simulink model "atrias_system_testing_delay"  (R2014a)
settings: Solver=FixedStepDiscrete  StartTime=0.0  StopTime=inf  FixedStep=sample_time  RelTol=1e-3
PreLoadFcn:
  | set_sampletime
PostLoadFcn:
  | set_sampletime
InitFcn:
  | sys_params
StartFcn:
  | set_sampletime
values from neighbouring files (symbols this model uses):
  A_lpf_velocity = 1 + B1_lpf_velocity + B2_lpf_velocity    [daq_params_osu.m]
  B1_lpf_velocity = -2*exp(-lpf_damping*fcut_velocity*sample_time)*cos(fcut_velocity*sample_time*sqrt(1-lpf_damping^2))    [daq_params_osu.m]
  B2_lpf_velocity = exp(-2*lpf_damping*fcut_velocity*sample_time)    [daq_params_osu.m]
  BOOM_MAX_ENCODER_TICKS = 2^17 - 1    (= 131071)    [daq_params_osu.m]
  BOOM_PITCH_CAL_VALUE_RAD = 0    [daq_params_osu.m]
  BOOM_PITCH_CAL_VALUE_TICKS = 43809    [daq_params_osu.m]
  BOOM_PITCH_ENCODER_RAD_PER_TICK = -2*pi / (2^17 * 2)    (= -2.39684498107e-05)    [daq_params_osu.m]
  BOOM_ROLL_CAL_VALUE_RAD = 0.1271    [daq_params_osu.m]
  BOOM_ROLL_CAL_VALUE_TICKS = 9318    [daq_params_osu.m]
  BOOM_ROLL_ENCODER_RAD_PER_TICK = 2*pi / (2^17 * 7)    (= 6.84812851735e-06)    [daq_params_osu.m]
  BOOM_YAW_ENCODER_RAD_PER_TICK = 2*pi / (2^17 * 9.6)    (= 4.9934270439e-06)    [daq_params_osu.m]
  CURRENT_LIMIT = 100    [daq_params_osu.m]
  fcut_smooth = 16*(2*pi)    (= 100.530964915)    [daq_params_osu.m]
  fcut_unwrap = 8*(2*pi)    (= 50.2654824574)    [daq_params_osu.m]
  gui_disable_cmd = 0    [daq_params_osu.m]
  gui_enable_cmd = 0    [daq_params_osu.m]
  gui_estop_cmd = 0    [daq_params_osu.m]
  gui_reset_cmd = 0    [daq_params_osu.m]
  HIP_ABS_ENCODER_RAD_PER_TICK = 2*pi / 2^13    (= 0.000766990393943)    [daq_params_osu.m]
  HIP_ABS_MAX_ENCODER_TICKS = 2^13 - 1    (= 8191)    [daq_params_osu.m]
  HIP_INC_ENCODER_RAD_PER_TICK = 2*pi / (2500 * 4 * 57)    (= 1.10231321179e-05)    [daq_params_osu.m]
  HIP_INC_MAX_ENCODER_TICKS = 2^16 - 1    (= 65535)    [daq_params_osu.m]
  HIP_MOTOR_CONSTANT = 0.184    [daq_params_osu.m]
  HIP_MTR_GEAR_RATIO = 57    [daq_params_osu.m]
  HIP_MTR_MAX_TORQUE = MTR_HIP_MAX_CURRENT*HIP_MOTOR_CONSTANT*HIP_MTR_GEAR_RATIO    (= 629.28)    [daq_params_osu.m]
  INC_ENC_DIRS = -[ LEG1_MOTOR_A_DIRECTION ... (first row only)    [daq_params_osu.m]
  INC_ENC_RAD_PER_TICK = 2*pi/14000/LEG_MTR_GEAR_RATIO    (= 8.97597901026e-06)    [daq_params_osu.m]
  k_sea = 4118    [sys_params.m]
  LEFT_HIP_CALIB_POS = 0    [daq_params_osu.m]
  LEFT_HIP_CALIB_VAL = 7192 - 2^13    (= -1000)    [daq_params_osu.m]
  LEFT_MOTOR_HIP_DIRECTION = -1.0    (= -1)    [daq_params_osu.m]
  LEG1_LEG_A_CALIB_VAL = 265417675    [daq_params_osu.m]
  LEG1_LEG_A_RAD_PER_CNT = -9.8039216e-09    [daq_params_osu.m]
  LEG1_LEG_B_CALIB_VAL = 175319150    [daq_params_osu.m]
  LEG1_LEG_B_RAD_PER_CNT = -9.8039216e-09    [daq_params_osu.m]
  LEG1_MOTOR_A_DIRECTION = -1.0    (= -1)    [daq_params_osu.m]
  LEG1_MOTOR_B_DIRECTION = -1.0    (= -1)    [daq_params_osu.m]
  LEG1_TRAN_A_CALIB_VAL = 143046540    [daq_params_osu.m]
  LEG1_TRAN_A_RAD_PER_CNT = 9.8039216e-09    [daq_params_osu.m]
  LEG1_TRAN_B_CALIB_VAL = 142356572    [daq_params_osu.m]
  LEG1_TRAN_B_RAD_PER_CNT = -9.8039216e-09    [daq_params_osu.m]
  LEG2_LEG_A_CALIB_VAL = 264357825    [daq_params_osu.m]
  LEG2_LEG_A_RAD_PER_CNT = -9.8039216e-09    [daq_params_osu.m]
  LEG2_LEG_B_CALIB_VAL = 261444054    [daq_params_osu.m]
  LEG2_LEG_B_RAD_PER_CNT = 9.8039216e-09    [daq_params_osu.m]
  LEG2_MOTOR_A_DIRECTION = 1.0    (= 1)    [daq_params_osu.m]
  LEG2_MOTOR_B_DIRECTION = 1.0    (= 1)    [daq_params_osu.m]
  LEG2_TRAN_A_CALIB_VAL = 142300933    [daq_params_osu.m]
  LEG2_TRAN_A_RAD_PER_CNT = 9.8039216e-09    [daq_params_osu.m]
  LEG2_TRAN_B_CALIB_VAL = 142287413    [daq_params_osu.m]
  LEG2_TRAN_B_RAD_PER_CNT = -9.8039216e-09    [daq_params_osu.m]
  LEG_A_CALIB_LOC = pi + 0.305432619099008    (= 3.44702527269)    [daq_params_osu.m]
  LEG_B_CALIB_LOC = pi - 0.305432619099008    (= 2.83616003449)    [daq_params_osu.m]
  LEG_MOTOR_CONSTANT = 0.119    [daq_params_osu.m]
  LEG_MTR_GEAR_RATIO = 50    [daq_params_osu.m]
  LEG_MTR_MAX_TORQUE = MTR_MAX_CURRENT*LEG_MOTOR_CONSTANT*LEG_MTR_GEAR_RATIO    (= 922.25)    [daq_params_osu.m]
  max_encoder_velocity = 200    [daq_params_osu.m]
  MEDULLA_ADC_MAX_VOLTS = 2.70    (= 2.7)    [daq_params_osu.m]
  MEDULLA_ADC_OFFSET_COUNTS = 172    [daq_params_osu.m]
  MEDULLA_STATE_ERROR = 5    [daq_params_osu.m]
  MEDULLA_STATE_HALT = 4    [daq_params_osu.m]
  MEDULLA_STATE_IDLE = 0    [daq_params_osu.m]
  MEDULLA_STATE_RESET = 6    [daq_params_osu.m]
  MEDULLA_STATE_RUN = 2    [daq_params_osu.m]
  MEDULLA_TIMER_FREQ = 32e6    (= 32000000)    [daq_params_osu.m]
  MOTOR_POSITION_LIMITS_LOWER = [2.5; 1.4; 0.4]    [daq_params_osu.m]
  MOTOR_POSITION_LIMITS_UPPER = [4.9; 3.8; 2.5]    [daq_params_osu.m]
  MTR_HIP_MAX_CURRENT = 60.0    (= 60)    [daq_params_osu.m]
  MTR_MAX_CONT_CURRENT = 100.0    (= 100)    [daq_params_osu.m]
  MTR_MAX_COUNT = 19900    [daq_params_osu.m]
  MTR_MAX_CURRENT = 155.0    (= 155)    [daq_params_osu.m]
  nom_sample_time = 0.001    [sys_params.m]
  RIGHT_HIP_CALIB_POS = 0    [daq_params_osu.m]
  RIGHT_HIP_CALIB_VAL = 1091    [daq_params_osu.m]
  RIGHT_MOTOR_HIP_DIRECTION = 1.0    (= 1)    [daq_params_osu.m]
  sample_time = 1/update_freq    (= 0.001)    [daq_params_osu.m]
  sensor_start_time = 8    [daq_params_osu.m]
undefined symbols (not defined in the file or in its folder): max_sensor_velocity
libraries: xpcethercatlib x196, simulink x50, slrtlib x4, dspswit3 x1
(part 1 of 4)
settings Model: xpc_rtwmakecfg_data=_xpcethercatlib_  SimulationMode=external  BufferReuse=off  Creator=wmartin  LastModifiedBy=drl
settings SolverCC: EnableConcurrentExecution=on
settings DataIOCC: MaxDataPoints=1000000000  SaveFormat=StructureWithTime  SaveOutput=off  SaveTime=off
settings OptimizationCC: BlockReduction=off  OptimizeBlockIOStorage=off  BufferReuse=off  GlobalBufferReuse=off  ExpressionFolding=off  ExpressionDepthLimit=2147483647  LocalBlockOutputs=off  SimCompilerOptimization=On
settings DebuggingCC: UnderspecifiedInitializationDetection=Classic  StateNameClashWarn=warning
settings HardwareCC: ProdIntDivRoundTo=Zero  ProdEndianess=LittleEndian  ProdHWDeviceType=Generic->32-bit x86 compatible
settings ModelReferenceCC: EnableParallelModelReferenceBuilds=on  ModelReferenceNumInstancesAllowed=Single  ModelReferenceMinAlgLoopOccurrences=on
settings RTWCC: SystemTargetFile=slrt.tlc  TemplateMakefile=slrt_default_tmf  Description=Simulink Real-Time  RTWVerbose=off  ProcessScript=slrt_make_rtw_hook  RTWCompilerOptimization=On
settings SimulinkRealTimeCC: GeneratePreprocessorConditionals=Disable all  EnableShiftOperators=on  RL32LogBufSizeModifier=100000000

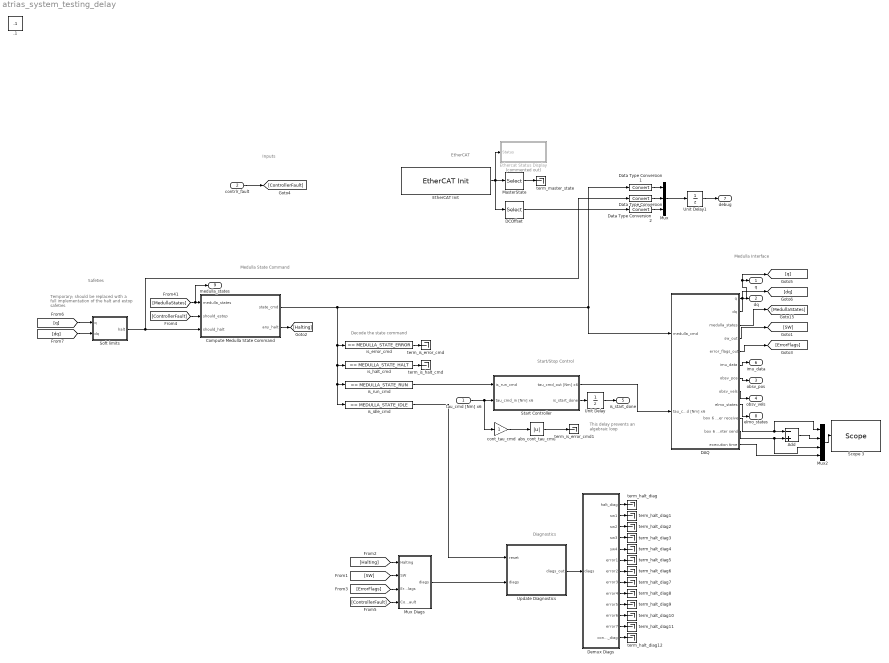
== system atrias_system_testing_delay ==
  note: Decode the state command
  note: Medulla Interface
  note: Medulla State Command
  note: Diagnostics
  note: EtherCAT
  note: Start/Stop Control
  note: Inputs
  note: Safeties
  note: Temporary; should be replaced with
      | a full implementation of the halt
      | and estop safeties
  note: This delay prevents
      | an algebraic loop
  tau_cmd [Nm] x6 : Inport
  contrlr_fault : Inport  Port=2  OutDataTypeStr=boolean
  Add : Sum  Inputs=-+
  Compute Medulla State Command : MATLAB Function  TreatAsAtomicUnit=on
  DAQ : Subsystem
  DCOffset : Selector  InputPortWidth=6  Indices=[4]
  Data Type Conversion : DataTypeConversion
  Data Type Conversion1 : DataTypeConversion
  Data Type Conversion2 : DataTypeConversion
  Demux Diags : MATLAB Function  TreatAsAtomicUnit=on
  EtherCAT Init : xpcethercatlib/EtherCAT Init   Priority=0  config_file=C:\Users\drl\Documents\MATLAB\7_medullas_4_elmos.xml  device_id=0  pci_bus=4  pci_slot=0  enaDebug=off  enaDC=on  errLink=off  masterDbg=off  stateChgDbg=off  baseClock=off  masterCfg=off  logFile='E:\dbglog.txt'  sample_time=0.001000
  Ethercat Status Display : Subsystem  Commented=on
  MasterState : Selector  InputPortWidth=6  Indices=[2]
  Mux : Mux  Inputs=3
  Mux Diags : MATLAB Function  TreatAsAtomicUnit=on
  Mux2 : Mux
  Scope 3 : slrtlib/Displays and Logging/Scope   scopeno=1  scopetype=Target  autostart=on  viewmode=Numerical  formatstr='%15.6f'  grid=on  ylimits=[0,0]  nosamples=100  noprepostsamples=0  interleave=1  triggermode=FreeRun  triggersignal=1  trigsignalfromport=off  triggerlevel=0.0  triggerslope=Either  triggerscope=1  triggersample=0  filename=data.dat  mode=Lazy  writesize=512  autorestart=off  dynamicfilemode=off  maxwritefilesize=512*1024^2
  Soft limits : MATLAB Function  TreatAsAtomicUnit=on
  Start Controller : Subsystem
  Unit Delay : UnitDelay  SampleTime=-1
  Unit Delay1 : UnitDelay  SampleTime=-1
  Update Diagnostics : MATLAB Function  TreatAsAtomicUnit=on
  abs_cont_tau_cmd : Abs
  cont_tau_cmd : Gain
  is_error_cmd : simulink/Logic and Bit Operations/Compare To Constant  relop===  const=MEDULLA_STATE_ERROR  OutDataTypeStr=boolean
  is_halt_cmd : simulink/Logic and Bit Operations/Compare To Constant  relop===  const=MEDULLA_STATE_HALT  OutDataTypeStr=boolean
  is_idle_cmd : simulink/Logic and Bit Operations/Compare To Constant  relop===  const=MEDULLA_STATE_IDLE  OutDataTypeStr=boolean
  is_run_cmd : simulink/Logic and Bit Operations/Compare To Constant  relop===  const=MEDULLA_STATE_RUN  OutDataTypeStr=boolean
  term_halt_diag{,1..12} (13 alike) : Terminator
  term_is_error_cmd : Terminator
  term_is_error_cmd1 : Terminator
  term_is_halt_cmd : Terminator
  term_master_state : Terminator
  q : Outport
  dq : Outport  Port=2
  obsv_pos : Outport  Port=3
  obsv_vels : Outport  Port=4
  is_start_done : Outport  Port=5
  imu_data : Outport  Port=6
  debug : Outport  Port=7
  elmo_states : Outport  Port=8
  medulla_states : Outport  Port=9
  .1 : Constant  IOType=siggen  Value=.1
  wires:
  MasterState/1 -> term_master_state/1
  DAQ/1(q) -> [q], q/1
  DAQ/2(dq) -> [dq], dq/1
  DAQ/3(medulla_states) -> [MedullaStates]
  [MedullaStates] -> medulla_states/1, Compute Medulla State Command/1(medulla_states)
  Compute Medulla State Command/2(any_halt) -> [Halting]
  Update Diagnostics/1(diags_out) -> Demux Diags/1(diags)
  is_halt_cmd/1 -> term_is_halt_cmd/1
  is_error_cmd/1 -> term_is_error_cmd/1
  tau_cmd [Nm] x6/1 -> cont_tau_cmd/1, Start Controller/2(tau_cmd_in [Nm] x6)
  is_run_cmd/1 -> Start Controller/1(is_run_cmd)
  Start Controller/1(tau_cmd_out [Nm] x6) -> DAQ/2(tau_cmd [Nm] x6)
  is_idle_cmd/1 -> Update Diagnostics/1(reset)
  DAQ/4(sw_out) -> [SW]
  Mux Diags/1(diags) -> Update Diagnostics/2(diags)
  [Halting] -> Mux Diags/1(Halting)
  [SW] -> Mux Diags/2(SW)
  Demux Diags/2(sw1) -> term_halt_diag1/1
  Demux Diags/5(sw4) -> term_halt_diag4/1
  Demux Diags/4(sw3) -> term_halt_diag3/1
  Demux Diags/3(sw2) -> term_halt_diag2/1
  DAQ/5(error_flags_out) -> [ErrorFlags]
  [ErrorFlags] -> Mux Diags/3(ErrorFlags)
  Demux Diags/1(halt_diag) -> term_halt_diag/1
  Demux Diags/12(error7) -> term_halt_diag11/1
  Demux Diags/11(error6) -> term_halt_diag10/1
  Demux Diags/10(error5) -> term_halt_diag9/1
  Demux Diags/9(error4) -> term_halt_diag8/1
  Demux Diags/8(error3) -> term_halt_diag7/1
  Demux Diags/7(error2) -> term_halt_diag6/1
  Demux Diags/6(error1) -> term_halt_diag5/1
  abs_cont_tau_cmd/1 -> term_is_error_cmd1/1
  DAQ/8(obsv_vels) -> obsv_vels/1
  Start Controller/2(is_start_done) -> Unit Delay/1
  DAQ/6(imu_data) -> imu_data/1
  DAQ/7(obsv_pos) -> obsv_pos/1
  contrlr_fault/1 -> [ControllerFault]
  [ControllerFault] -> Compute Medulla State Command/2(should_estop)
  [ControllerFault] -> Mux Diags/4(ControllerFault)
  Demux Diags/13(contrlr_fault_diag) -> term_halt_diag12/1
  Unit Delay/1 -> is_start_done/1
  [q] -> Soft limits/1(q)
  [dq] -> Soft limits/2(dq)
  Soft limits/1(halt) -> Data Type Conversion/1, Compute Medulla State Command/3(should_halt)
  Unit Delay1/1 -> debug/1
  Mux/1 -> Unit Delay1/1
  Data Type Conversion/1 -> Mux/2
  Data Type Conversion1/1 -> Mux/1
  DCOffset/1 -> Data Type Conversion2/1
  Data Type Conversion2/1 -> Mux/3
  DAQ/9(elmo_states) -> elmo_states/1
  EtherCAT Init/1 -> MasterState/1, DCOffset/1, Ethercat Status Display/1(Status)
  Compute Medulla State Command/1(state_cmd) -> is_run_cmd/1, is_idle_cmd/1, is_halt_cmd/1, is_error_cmd/1, Data Type Conversion1/1, DAQ/1(medulla_cmd)
  cont_tau_cmd/1 -> abs_cont_tau_cmd/1
  DAQ/10(box 6 counter receive) -> Mux2/1, Add/1
  DAQ/11(box 6 counter send) -> Mux2/3, Add/2
  Add/1 -> Mux2/2
  Mux2/1 -> Scope 3/1
  DAQ/12(execution time) -> Mux2/4

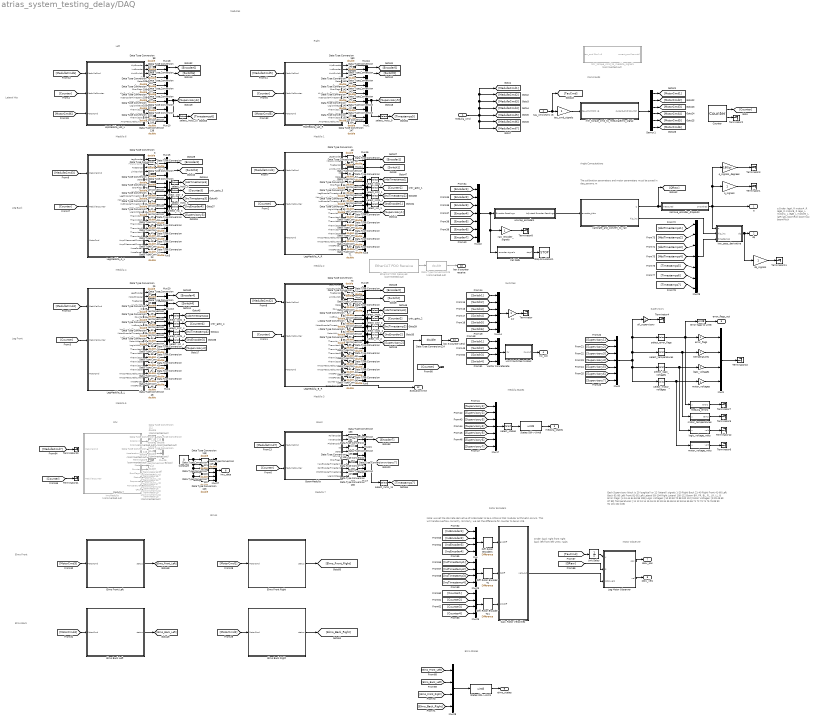
== system atrias_system_testing_delay/DAQ ==
  note: Order:
      |
      | back right
      | front right
      | back left
      | front left
      |
      | Units: rad/s
  note: Left
  note: The calibration parameters and motor parameters
      | must be saved in daq_params.m
  note: Right
  note: Lateral Hip
  note: Leg Back
  note: Leg Front
  note: Boom
  note: Medullas
  note: Angle Computations
  note: Commands
  note: Switches
  note: Supervisory
  note: Medulla 2
  note: Medulla 3
  note: Medulla 5
  note: Medulla 4
  note: Medulla 6
  note: Medulla 1
  note: Medulla 7
  note: Each Supervisory block is 20 (sagittal) or 12 (lateral) signals
      | 1-20      Right Back
      | 21-40     Right Front
      | 41-60     Left Back
      | 61-80     Left Front
      | 81-92     Left Lateral
      | 93-104    Right Lateral
      | 105-112   Boom
      |
      | BR, FR, BL, FL, LR, LL, B
      | Error Flags: [4 24 44 64 84 96 108]
      | Logic Voltages: [10 30 50 70 88 100 112]
      | Motor Voltages: [9 29 49 69 87 99]
      | Temperatures: [11 12 13 14 15 16 31 32 33 34 35 36 51 52 53 54 55 56 71 72 73 74 75 76 89 90 91 101 102 103]
  note: q Order:
      |
      | legA_R
      | motorA_R
      | legB_R
      | motorB_R
      |
      | legA_L
      | motorA_L
      | legB_L
      | motorB_L
      |
      | latR
      | latL
      |
      | boomRoll
      | boomYaw
      | boomPitch
  note: Medulla States
  note: Rotor Encoders
  note: Note: we set the discrete derivative of IncEncoder to be a int16 so that modular arithmetic occurs.
      | This will handle overflow correctly. Similarly, we set the difference for counter to be an int8.
  note: Medulla 7
  note: IMU
  note: Motor Observer
  note: Elmos
  note: Elmo Front
  note: Elmo Back
  note: Elmo States
  medulla_cmd : Inport
  tau_cmd [Nm] x6 : Inport  Port=2  OutDataTypeStr=double  PortDimensions=6  SampleTime=0
  BoomMedulla : Subsystem
  Calc. Rotor Velocities : MATLAB Function  TreatAsAtomicUnit=on
  Constant : Constant  Value=0
  Counter : dspswit3/Counter  Direction=Up  CountEvent=Free running  CounterSize=User defined  MaxCount=255  InitialCount=0  Output=Count and Hit  HitValue=32  ResetInput=off  SamplesPerFrame=1  Ts=.001  CntDtype=double  HitDtype=Logical
  Data Type Conversion{1..111,118..124,127..151,157} (144 alike) : DataTypeConversion  OutDataTypeStr=double
  Data Type Conversion{112..117,125} (7 alike) : DataTypeConversion  Commented=on  OutDataTypeStr=double
  Demux1 : Demux  Outputs=6
  Diff. Rotor Encoder Ts : simulink/Discrete/Difference  ICPrevInput=0.0  InputProcessing=Inherited  OutMin=[]  OutMax=[]  OutDataType=fixdt(1, 16)  OutScaling=2^-10  RndMeth=Nearest  DoSatur=off
  Diff. Rotor Encoder Ts1 : simulink/Discrete/Difference  ICPrevInput=0.0  InputProcessing=Inherited  OutMin=[]  OutMax=[]  OutDataTypeStr=int16  OutputDataTypeScalingMode=int16  OutDataType=fixdt(1, 16)  OutScaling=2^-10  RndMeth=Nearest  DoSatur=off
  Diff. Rotor Encoders : simulink/Discrete/Difference  ICPrevInput=0.0  InputProcessing=Inherited  OutMin=[]  OutMax=[]  OutDataTypeStr=int32  OutputDataTypeScalingMode=int32  OutDataType=fixdt(1, 16)  OutScaling=2^-10  RndMeth=Nearest  DoSatur=off
  Elmo Back Left : Subsystem
  Elmo Back Right : Subsystem
  Elmo Front Left : Subsystem
  Elmo Front Right : Subsystem
  Error flags to uint8 : DataTypeConversion  OutDataTypeStr=uint8
  EtherCAT PDO Receive8 : xpcethercatlib/EtherCAT PDO Receive  Priority=2  Commented=on  sig_name=Box 6 (ATRIAS 2.1 Leg (Medulla 1.5)).Motor Encoder.Motor Encoder  sig_offset=1648  sig_type=uint32  type_size=32  sig_dim=1  device_id=0  sample_time=0.001
  Fail Safe : Subsystem
  HipMedulla_Lat_L : Subsystem
  HipMedulla_Lat_R : Subsystem
  ImuMedulla : Subsystem  Commented=on
  Leg Motor Observer : MATLAB Function  TreatAsAtomicUnit=on
  LegMedulla_A_L : Subsystem
  LegMedulla_A_R : Subsystem
  LegMedulla_B_L : Subsystem
  LegMedulla_B_R : Subsystem
  Limit Switches to Bool : MATLAB Function  TreatAsAtomicUnit=on
  Mux{,9,23,25,28} (5 alike) : Mux
  Mux1 : Mux  Inputs=12
  Mux10 : Mux  Inputs=12
  Mux{2,11..13,15..16,18..20,24} (10 alike) : Mux  Inputs=2
  Mux14 : Mux  Inputs=6
  Mux{8,17,22,29} (4 alike) : Mux  Inputs=7
  Mux21 : Mux  Inputs=3
  Mux26 : Mux  Commented=on  Inputs=6
  Mux27 : Mux  Inputs=6
  Mux{3..6} (4 alike) : Mux  Inputs=20
  Mux7 : Mux  Inputs=8
  States Dbl->Uint1 : DataTypeConversion  OutDataTypeStr=uint8
  States Dbl->Uint8 : DataTypeConversion  OutDataTypeStr=uint8
  Stop Simulation1 : Stop
  Terminator{,1..8,10..12,20..21} (14 alike) : Terminator
  Terminator{9,13..19} (8 alike) : Terminator  Commented=on
  Unit Delay : UnitDelay  SampleTime=-1
  Vector Concatenate : Concatenate  NumInputs=4
  all_supervisory : Gain
  calibrate_and_convert_to_rad : Subsystem
  dq_signals : Gain
  error_flags : Gain
  logic_voltage_volts : MATLAB Function  TreatAsAtomicUnit=on
  logic_voltages : Gain
  low_pass_derivative : Subsystem
  medulla_errors : MATLAB Function  TreatAsAtomicUnit=on
  motor_temperatures : MATLAB Function  TreatAsAtomicUnit=on
  motor_voltage_volts : MATLAB Function  TreatAsAtomicUnit=on
  motor_voltages : Gain
  mtr_torque_cmd_to_medulla/elmo_signal : Subsystem
  mtr_torque_cmd_to_medulla_signal1 : Subsystem  Commented=on
  q_signals : Gain
  q_signals_degrees : Gain  Gain=180/pi
  raw_encoder_signals : Gain
  remove_encoder_dropouts : Subsystem
  select_cntr_{1..4} (4 alike) : Selector  InputPortWidth=20  Indices=3
  select_error_flags : Selector  InputPortWidth=112  Indices=[4 24 44 64 84 96 108]
  select_inc_{1..4} (4 alike) : Selector  InputPortWidth=20  Indices=5
  select_incts_{1..4} (4 alike) : Selector  InputPortWidth=20  Indices=8
  select_incts_10 : Selector  InputPortWidth=12  Indices=[6]
  select_incts_11 : Selector  InputPortWidth=8  Indices=[5 6 7]
  select_incts_{5..8} (4 alike) : Selector  InputPortWidth=20  Indices=[6 7]
  select_incts_9 : Selector  InputPortWidth=12  Indices=[6]
  select_logic_voltages : Selector  InputPortWidth=112  Indices=[10 30 50 70 88 100 112]
  select_motor_voltages : Selector  InputPortWidth=112  Indices=[9 29 49 69 87 99]
  select_states : Selector  InputPortWidth=112  Indices=[2 22 42 62 82 94 106]
  select_temperatures : Selector  InputPortWidth=112  Indices=[11 12 13 14 15 16 31 32 33 34 35 36 51 52 53 54 55 56 71 72 73 74 75 76 89 90 91 101 102 103]
  sw : Gain
  tau_cmd_signals : Gain
  temperatures : Gain
  unwrap_encoders : Subsystem
  q : Outport  OutDataTypeStr=double  PortDimensions=13  SampleTime=[0.001,0]
  dq : Outport  Port=2  OutDataTypeStr=double  PortDimensions=13  SampleTime=[0.001,0]
  medulla_states : Outport  Port=3  OutDataTypeStr=uint8
  sw_out : Outport  Port=4
  error_flags_out : Outport  Port=5  OutDataTypeStr=uint8
  imu_data : Outport  Port=6
  obsv_pos : Outport  Port=7
  obsv_vels : Outport  Port=8
  elmo_states : Outport  Port=9  OutDataTypeStr=uint8
  box 6 counter receive : Outport  Port=10
  box 6 counter send : Outport  Port=11
  execution time : Outport  Port=12
  wires:
  BoomMedulla/11(LogicVoltage) -> Data Type Conversion136/1
  BoomMedulla/10(PitchEncoderTimestamp) -> Data Type Conversion137/1
  BoomMedulla/9(RollEncoderTimestamp) -> Data Type Conversion127/1
  BoomMedulla/8(YawEncoderTimestamp) -> Data Type Conversion129/1
  BoomMedulla/7(ErrorFlags) -> Data Type Conversion130/1
  BoomMedulla/6(Counter) -> Data Type Conversion128/1
  BoomMedulla/5(State) -> Data Type Conversion134/1
  BoomMedulla/4(ID) -> Data Type Conversion135/1
  BoomMedulla/3(PitchEncoder) -> Data Type Conversion131/1
  BoomMedulla/2(YawEncoder) -> Data Type Conversion132/1
  BoomMedulla/1(RollEncoder) -> Data Type Conversion133/1
  Data Type Conversion133/1 -> Mux21/1
  Data Type Conversion132/1 -> Mux21/2
  Data Type Conversion131/1 -> Mux21/3
  Data Type Conversion135/1 -> Mux7/1
  Data Type Conversion134/1 -> Mux7/2
  Data Type Conversion128/1 -> Mux7/3
  Data Type Conversion130/1 -> Mux7/4
  Data Type Conversion129/1 -> Mux7/5
  Data Type Conversion127/1 -> Mux7/6
  Data Type Conversion137/1 -> Mux7/7
  Data Type Conversion136/1 -> Mux7/8
  Data Type Conversion98/1 -> Mux18/1
  Data Type Conversion97/1 -> Mux18/2
  Data Type Conversion110/1 -> Mux10/1
  Data Type Conversion105/1 -> Mux10/2
  Data Type Conversion107/1 -> Mux10/3
  Data Type Conversion106/1 -> Mux10/4
  Data Type Conversion109/1 -> Mux10/5
  Data Type Conversion108/1 -> Mux10/6
  Data Type Conversion101/1 -> Mux10/7
  Data Type Conversion103/1 -> Mux10/8
  Data Type Conversion102/1 -> Mux10/9
  Data Type Conversion100/1 -> Mux10/10
  Data Type Conversion99/1 -> Mux10/11
  mtr_torque_cmd_to_medulla/elmo_signal/1(current_cmd [counts]) -> Demux1/1
  Data Type Conversion50/1 -> Mux16/2
  Data Type Conversion49/1 -> Mux16/1
  Data Type Conversion48/1 -> Mux4/20
  Data Type Conversion47/1 -> Mux4/19
  Data Type Conversion46/1 -> Mux4/18
  Data Type Conversion45/1 -> Mux4/17
  Data Type Conversion44/1 -> Mux4/16
  Data Type Conversion43/1 -> Mux4/15
  Data Type Conversion42/1 -> Mux4/14
  Data Type Conversion41/1 -> Mux4/13
  Data Type Conversion40/1 -> Mux4/12
  Data Type Conversion39/1 -> Mux4/11
  Data Type Conversion38/1 -> Mux4/10
  Data Type Conversion37/1 -> Mux4/9
  Data Type Conversion36/1 -> Mux4/8
  Data Type Conversion35/1 -> Mux4/7
  Data Type Conversion34/1 -> Mux4/6
  Data Type Conversion33/1 -> Mux4/5
  Data Type Conversion32/1 -> Mux4/4
  Data Type Conversion31/1 -> Mux4/3
  Data Type Conversion30/1 -> Mux4/2
  Data Type Conversion29/1 -> Mux4/1
  Data Type Conversion28/1 -> Mux13/2
  Data Type Conversion27/1 -> Mux13/1
  Data Type Conversion26/1 -> Mux20/2
  Data Type Conversion25/1 -> Mux20/1
  Data Type Conversion24/1 -> Mux3/20
  Data Type Conversion23/1 -> Mux3/19
  Data Type Conversion22/1 -> Mux3/18
  Data Type Conversion21/1 -> Mux3/17
  Data Type Conversion20/1 -> Mux3/16
  Data Type Conversion19/1 -> Mux3/15
  Data Type Conversion18/1 -> Mux3/14
  Data Type Conversion17/1 -> Mux3/13
  Data Type Conversion16/1 -> Mux3/12
  Data Type Conversion15/1 -> Mux3/11
  Data Type Conversion14/1 -> Mux3/10
  Data Type Conversion13/1 -> Mux3/9
  Data Type Conversion12/1 -> Mux3/8
  Data Type Conversion11/1 -> Mux3/7
  Data Type Conversion10/1 -> Mux3/6
  Data Type Conversion9/1 -> Mux3/5
  Data Type Conversion8/1 -> Mux3/4
  Data Type Conversion7/1 -> Mux3/3
  Data Type Conversion6/1 -> Mux3/2
  Data Type Conversion5/1 -> Mux3/1
  Data Type Conversion4/1 -> Mux2/2
  Data Type Conversion2/1 -> Mux2/1
  Data Type Conversion1/1 -> Mux15/2
  Data Type Conversion3/1 -> Mux15/1
  tau_cmd [Nm] x6/1 -> [TauCmd], tau_cmd_signals/1
  Data Type Conversion138/1 -> Mux10/12
  Data Type Conversion96/1 -> Mux6/20
  Data Type Conversion95/1 -> Mux6/19
  Data Type Conversion94/1 -> Mux6/18
  Data Type Conversion93/1 -> Mux6/17
  Data Type Conversion92/1 -> Mux6/16
  Data Type Conversion91/1 -> Mux6/15
  Data Type Conversion90/1 -> Mux6/14
  Data Type Conversion89/1 -> Mux6/13
  Data Type Conversion88/1 -> Mux6/12
  Data Type Conversion87/1 -> Mux6/11
  Data Type Conversion86/1 -> Mux6/10
  Data Type Conversion85/1 -> Mux6/9
  Data Type Conversion84/1 -> Mux6/8
  Data Type Conversion83/1 -> Mux6/7
  Data Type Conversion82/1 -> Mux6/6
  Data Type Conversion81/1 -> Mux6/5
  Data Type Conversion80/1 -> Mux6/4
  Data Type Conversion79/1 -> Mux6/3
  Data Type Conversion78/1 -> Mux6/2
  Data Type Conversion77/1 -> Mux6/1
  Data Type Conversion76/1 -> Mux12/2
  Data Type Conversion75/1 -> Mux12/1
  Data Type Conversion74/1 -> Mux19/2
  Data Type Conversion73/1 -> Mux19/1
  Data Type Conversion72/1 -> Mux5/20
  Data Type Conversion71/1 -> Mux5/19
  Data Type Conversion70/1 -> Mux5/18
  Data Type Conversion69/1 -> Mux5/17
  Data Type Conversion68/1 -> Mux5/16
  Data Type Conversion67/1 -> Mux5/15
  Data Type Conversion66/1 -> Mux5/14
  Data Type Conversion65/1 -> Mux5/13
  Data Type Conversion64/1 -> Mux5/12
  Data Type Conversion63/1 -> Mux5/11
  Data Type Conversion62/1 -> Mux5/10
  Data Type Conversion61/1 -> Mux5/9
  Data Type Conversion60/1 -> Mux5/8
  Data Type Conversion59/1 -> Mux5/7
  Data Type Conversion58/1 -> Mux5/6
  Data Type Conversion57/1 -> Mux5/5
  Data Type Conversion56/1 -> Mux5/4
  Data Type Conversion55/1 -> Mux5/3
  Data Type Conversion54/1 -> Mux5/2
  Data Type Conversion53/1 -> Mux5/1
  Data Type Conversion52/1 -> Mux11/2
  Data Type Conversion51/1 -> Mux11/1
  Counter/2 -> Terminator2/1
  Counter/1 -> [Counter]
  [Counter] -> BoomMedulla/2(MedullaCounter)
  [MedullaCmd7] -> BoomMedulla/1(MedullaCmd)
  Data Type Conversion157/1 -> [Switch6]
  [Switch1] -> Mux14/1
  [Switch2] -> Mux14/2
  [Switch3] -> Mux14/3
  [Switch4] -> Mux14/4
  [Switch5] -> Mux14/5
  [Switch6] -> Mux14/6
  low_pass_derivative/1(dq) -> dq_signals/1, dq/1
  Demux1/1 -> [MotorCmd1]
  Demux1/2 -> [MotorCmd2]
  Demux1/3 -> [MotorCmd3]
  Demux1/4 -> [MotorCmd4]
  Demux1/5 -> [MotorCmd5]
  Demux1/6 -> [MotorCmd6]
  Mux2/1 -> [Switch3]
  Mux3/1 -> select_incts_5/1, select_cntr_3/1, select_incts_3/1, select_inc_3/1, [Supervisory3]
  Mux4/1 -> [Supervisory4], select_incts_6/1, select_cntr_4/1, select_incts_4/1, select_inc_4/1
  Mux5/1 -> [Supervisory1], select_incts_8/1, select_cntr_1/1, select_incts_1/1, select_inc_1/1
  Mux6/1 -> select_incts_7/1, select_cntr_2/1, select_incts_2/1, select_inc_2/1, [Supervisory2]
  [Supervisory1] -> Mux8/1
  [Supervisory2] -> Mux8/2
  [Supervisory3] -> Mux8/3
  [Supervisory4] -> Mux8/4
  [Supervisory5] -> Mux8/5
  [Supervisory6] -> Mux8/6
  [Supervisory7] -> Mux8/7
  Mux11/1 -> [Switch1]
  Mux12/1 -> [Switch2]
  Mux13/1 -> [Switch4]
  Mux15/1 -> [Encoder3]
  Mux16/1 -> [Encoder1]
  Mux18/1 -> [Encoder6]
  Mux19/1 -> [Encoder2]
  Mux20/1 -> [Encoder4]
  Mux21/1 -> [Encoder7]
  [Encoder7] -> Mux22/7
  [Encoder6] -> Mux22/6
  [Encoder5] -> Mux22/5
  [Encoder4] -> Mux22/4
  [Encoder3] -> Mux22/3
  [Encoder2] -> Mux22/2
  [Encoder1] -> Mux22/1
  Mux22/1 -> unwrap_encoders/1(Encoder Readings), raw_encoder_signals/1, Fail Safe/1(encoder signals)
  Data Type Conversion150/1 -> Mux24/1
  Data Type Conversion149/1 -> Mux24/2
  Data Type Conversion146/1 -> Mux1/1
  Data Type Conversion141/1 -> Mux1/2
  Data Type Conversion143/1 -> Mux1/3
  Data Type Conversion142/1 -> Mux1/4
  Data Type Conversion145/1 -> Mux1/5
  Data Type Conversion144/1 -> Mux1/6
  Data Type Conversion111/1 -> Mux1/7
  Data Type Conversion140/1 -> Mux1/8
  Data Type Conversion139/1 -> Mux1/9
  Data Type Conversion104/1 -> Mux1/10
  Data Type Conversion151/1 -> Mux1/11
  Data Type Conversion147/1 -> Mux1/12
  Data Type Conversion148/1 -> [Switch5]
  Mux24/1 -> [Encoder5]
  q_signals/1 -> Terminator1/1
  tau_cmd_signals/1 -> mtr_torque_cmd_to_medulla/elmo_signal/1(tau_cmd [Nm] x6)
  Mux8/1 -> select_temperatures/1, select_error_flags/1, all_supervisory/1, select_motor_voltages/1, select_logic_voltages/1
  select_error_flags/1 -> error_flags/1, medulla_errors/1(u), Error flags to uint8/1
  select_temperatures/1 -> temperatures/1, motor_temperatures/1(u)
  select_logic_voltages/1 -> logic_voltage_volts/1(u), logic_voltages/1
  select_motor_voltages/1 -> motor_voltages/1, motor_voltage_volts/1(u)
  error_flags/1 -> Mux9/1
  temperatures/1 -> Mux9/2
  logic_voltages/1 -> Mux9/3
  motor_voltages/1 -> Mux9/4
  Mux9/1 -> Terminator10/1
  q_signals_degrees/1 -> Terminator3/1
  calibrate_and_convert_to_rad/1(q) -> [QRaw], remove_encoder_dropouts/1(measured)
  all_supervisory/1 -> Terminator4/1
  motor_temperatures/1(temp) -> Terminator5/1
  motor_voltage_volts/1(volt) -> Terminator6/1
  medulla_errors/1(errors) -> Terminator7/1
  remove_encoder_dropouts/1(smoothed) -> low_pass_derivative/1(q), q_signals/1, q_signals_degrees/1, q/1
  unwrap_encoders/1(Adjusted Encoder Readings) -> calibrate_and_convert_to_rad/1(encoder_ticks)
  dq_signals/1 -> Terminator11/1
  logic_voltage_volts/1(volt) -> Terminator12/1
  medulla_cmd/1 -> [MedullaCmd3], [MedullaCmd2], [MedullaCmd1], [MedullaCmd4], [MedullaCmd6], [MedullaCmd7], [MedullaCmd5]
  [Supervisory1] -> Mux17/1
  [Supervisory2] -> Mux17/2
  [Supervisory3] -> Mux17/3
  [Supervisory4] -> Mux17/4
  [Supervisory5] -> Mux17/5
  [Supervisory6] -> Mux17/6
  [Supervisory7] -> Mux17/7
  Mux17/1 -> select_states/1
  select_states/1 -> States Dbl->Uint8/1
  States Dbl->Uint8/1 -> medulla_states/1
  Mux14/1 -> sw/1
  sw/1 -> Terminator/1
  [Switch1] -> Vector Concatenate/1
  [Switch2] -> Vector Concatenate/2
  [Switch3] -> Vector Concatenate/3
  [Switch4] -> Vector Concatenate/4
  Vector Concatenate/1 -> Limit Switches to Bool/1(sw)
  Limit Switches to Bool/1(sw_out) -> sw_out/1
  Error flags to uint8/1 -> error_flags_out/1
  select_inc_1/1 -> [IncEncoder1]
  select_inc_2/1 -> [IncEncoder2]
  select_inc_4/1 -> [IncEncoder3]
  select_inc_3/1 -> [IncEncoder4]
  select_incts_1/1 -> [IncTimestamp1]
  select_incts_2/1 -> [IncTimestamp2]
  select_incts_3/1 -> [IncTimestamp3]
  select_incts_4/1 -> [IncTimestamp4]
  [IncEncoder1] -> Mux/1
  [IncEncoder2] -> Mux/2
  [IncEncoder3] -> Mux/3
  [IncEncoder4] -> Mux/4
  [IncTimestamp1] -> Mux23/1
  [IncTimestamp2] -> Mux23/2
  [IncTimestamp3] -> Mux23/3
  [IncTimestamp4] -> Mux23/4
  Mux/1 -> Diff. Rotor Encoders/1
  Mux23/1 -> Diff. Rotor Encoder Ts/1
  Diff. Rotor Encoder Ts/1 -> Calc. Rotor Velocities/2(tsdiff)
  Diff. Rotor Encoders/1 -> Calc. Rotor Velocities/1(encdiff)
  Calc. Rotor Velocities/1(vels_out) -> Leg Motor Observer/3(rotor_vels)
  select_cntr_1/1 -> [Counter1]
  select_cntr_2/1 -> [Counter2]
  select_cntr_3/1 -> [Counter3]
  select_cntr_4/1 -> [Counter4]
  [Counter1] -> Mux25/1
  [Counter2] -> Mux25/2
  [Counter3] -> Mux25/3
  [Counter4] -> Mux25/4
  Mux25/1 -> Diff. Rotor Encoder Ts1/1
  Diff. Rotor Encoder Ts1/1 -> Calc. Rotor Velocities/3(cntrdiff)
  ImuMedulla/3(RotationZ) -> Data Type Conversion114/1
  ImuMedulla/2(RotationX) -> Data Type Conversion113/1
  ImuMedulla/1(RotationY) -> Data Type Conversion112/1
  ImuMedulla/4(AccelerationX) -> Data Type Conversion115/1
  ImuMedulla/5(AccelerationY) -> Data Type Conversion116/1
  ImuMedulla/6(AccelerationZ) -> Data Type Conversion117/1
  Data Type Conversion112/1 -> Mux26/1
  Data Type Conversion113/1 -> Mux26/2
  Data Type Conversion114/1 -> Mux26/3
  ImuMedulla/7(ID) -> Terminator9/1
  ImuMedulla/8(State) -> Terminator13/1
  ImuMedulla/14(CRC) -> Terminator18/1
  ImuMedulla/13(Temperature) -> Terminator19/1
  ImuMedulla/12(Sequence) -> Terminator16/1
  ImuMedulla/11(Status) -> Terminator17/1
  ImuMedulla/10(ErrorFlags) -> Terminator14/1
  ImuMedulla/9(Counter) -> Terminator15/1
  Data Type Conversion117/1 -> Mux26/6
  Data Type Conversion116/1 -> Mux26/5
  Data Type Conversion115/1 -> Mux26/4
  Mux26/1 -> ?
  [QRaw] -> Leg Motor Observer/2(q)
  Leg Motor Observer/2(vel) -> obsv_vels/1
  Leg Motor Observer/1(pos) -> obsv_pos/1
  Unit Delay/1 -> Leg Motor Observer/1(u)
  [TauCmd] -> Unit Delay/1
  Data Type Conversion118/1 -> Mux27/1
  Data Type Conversion119/1 -> Mux27/2
  Data Type Conversion120/1 -> Mux27/3
  Data Type Conversion123/1 -> Mux27/6
  Data Type Conversion122/1 -> Mux27/5
  Data Type Conversion121/1 -> Mux27/4
  Mux27/1 -> imu_data/1
  Constant/1 -> Data Type Conversion123/1, Data Type Conversion122/1, Data Type Conversion121/1, Data Type Conversion120/1, Data Type Conversion119/1, Data Type Conversion118/1
  [MedullaCmd7] -> Terminator20/1
  [Counter] -> Terminator21/1
  Fail Safe/1(stop?) -> Stop Simulation1/1
  raw_encoder_signals/1 -> Terminator8/1
  select_incts_5/1 -> [AbsTimestamps3]
  select_incts_6/1 -> [AbsTimestamps4]
  select_incts_7/1 -> [AbsTimestamps2]
  select_incts_8/1 -> [AbsTimestamps1]
  calibrate_and_convert_to_rad/2(hip_inc) -> low_pass_derivative/2(hip_inc)
  [Elmo_Front_Left] -> Mux28/1
  States Dbl->Uint1/1 -> elmo_states/1
  Mux28/1 -> States Dbl->Uint1/1
  [Elmo_Back_Left] -> Mux28/2
  [Elmo_Front_Right] -> Mux28/3
  [Elmo_Back_Right] -> Mux28/4
  [AbsTimestamps1] -> Mux29/1
  [AbsTimestamps2] -> Mux29/2
  [AbsTimestamps3] -> Mux29/3
  [AbsTimestamps4] -> Mux29/4
  select_incts_9/1 -> [Timestamps5]
  Mux1/1 -> select_incts_9/1, [Supervisory5]
  select_incts_10/1 -> [Timestamps6]
  Mux10/1 -> select_incts_10/1, [Supervisory6]
  [Timestamps5] -> Mux29/5
  [Timestamps6] -> Mux29/6
  Mux29/1 -> low_pass_derivative/3(timestamps)
  select_incts_11/1 -> [Timestamps7]
  Mux7/1 -> select_incts_11/1, [Supervisory7]
  [Timestamps7] -> Mux29/7
  HipMedulla_Lat_L/1(HipEncoder) -> Data Type Conversion98/1
  HipMedulla_Lat_L/2(IncEncoder) -> Data Type Conversion97/1
  HipMedulla_Lat_L/3(LimitSwitch) -> Data Type Conversion157/1
  HipMedulla_Lat_L/4(ID) -> Data Type Conversion110/1
  HipMedulla_Lat_L/5(State) -> Data Type Conversion105/1
  HipMedulla_Lat_L/6(Counter) -> Data Type Conversion107/1
  HipMedulla_Lat_L/7(ErrorFlags) -> Data Type Conversion106/1
  HipMedulla_Lat_L/8(HipEncoderTimestamp) -> Data Type Conversion109/1
  HipMedulla_Lat_L/9(IncEncoderTimestamp) -> Data Type Conversion108/1
  HipMedulla_Lat_L/10(MotorVoltage) -> Data Type Conversion101/1
  HipMedulla_Lat_L/11(LogicVoltage) -> Data Type Conversion103/1
  HipMedulla_Lat_L/12(Thermistor0) -> Data Type Conversion102/1
  HipMedulla_Lat_L/13(Thermistor1) -> Data Type Conversion100/1
  HipMedulla_Lat_L/14(Thermistor2) -> Data Type Conversion99/1
  HipMedulla_Lat_L/15(AmpMeasuredCurrent) -> Data Type Conversion138/1
  [MedullaCmd6] -> HipMedulla_Lat_L/1(MedullaCmd)
  [Counter] -> HipMedulla_Lat_L/2(MedullaCounter)
  [MotorCmd6] -> HipMedulla_Lat_L/3(MotorCmd)
  [MedullaCmd5] -> HipMedulla_Lat_R/1(MedullaCmd)
  [Counter] -> HipMedulla_Lat_R/2(MedullaCounter)
  [MotorCmd5] -> HipMedulla_Lat_R/3(MotorCmd)
  HipMedulla_Lat_R/1(HipEncoder) -> Data Type Conversion150/1
  HipMedulla_Lat_R/2(IncEncoder) -> Data Type Conversion149/1
  HipMedulla_Lat_R/3(LimitSwitch) -> Data Type Conversion148/1
  HipMedulla_Lat_R/4(ID) -> Data Type Conversion146/1
  HipMedulla_Lat_R/5(State) -> Data Type Conversion141/1
  HipMedulla_Lat_R/6(Counter) -> Data Type Conversion143/1
  HipMedulla_Lat_R/7(ErrorFlags) -> Data Type Conversion142/1
  HipMedulla_Lat_R/8(HipEncoderTimestamp) -> Data Type Conversion145/1
  HipMedulla_Lat_R/9(IncEncoderTimestamp) -> Data Type Conversion144/1
  HipMedulla_Lat_R/10(MotorVoltage) -> Data Type Conversion111/1
  HipMedulla_Lat_R/11(LogicVoltage) -> Data Type Conversion140/1
  HipMedulla_Lat_R/12(Thermistor0) -> Data Type Conversion139/1
  HipMedulla_Lat_R/13(Thermistor1) -> Data Type Conversion104/1
  HipMedulla_Lat_R/14(Thermistor2) -> Data Type Conversion151/1
  HipMedulla_Lat_R/15(AmpMeasuredCurrent) -> Data Type Conversion147/1
  LegMedulla_A_L/1(LegEncoder) -> Data Type Conversion3/1
  LegMedulla_A_L/2(MotorEncoder) -> Data Type Conversion1/1
  LegMedulla_A_L/3(ToeSensor) -> Data Type Conversion2/1
  LegMedulla_A_L/4(LimitSwitch) -> Data Type Conversion4/1
  LegMedulla_A_L/5(ID) -> Data Type Conversion5/1
  LegMedulla_A_L/6(State) -> Data Type Conversion6/1
  LegMedulla_A_L/7(Counter) -> Data Type Conversion7/1
  LegMedulla_A_L/8(ErrorFlags) -> Data Type Conversion8/1
  LegMedulla_A_L/9(IncEncoder) -> Data Type Conversion9/1
  LegMedulla_A_L/10(LegEncoderTimestamp) -> Data Type Conversion10/1
  LegMedulla_A_L/11(MotorEncoderTimestamp) -> Data Type Conversion11/1
  LegMedulla_A_L/12(IncEncoderTimestamp) -> Data Type Conversion12/1
  LegMedulla_A_L/13(MotorVoltage) -> Data Type Conversion13/1
  LegMedulla_A_L/14(LogicVoltage) -> Data Type Conversion14/1
  LegMedulla_A_L/15(Thermistor0) -> Data Type Conversion15/1
  LegMedulla_A_L/16(Thermistor1) -> Data Type Conversion16/1
  LegMedulla_A_L/17(Thermistor2) -> Data Type Conversion17/1
  LegMedulla_A_L/18(Thermistor3) -> Data Type Conversion18/1
  LegMedulla_A_L/19(Thermistor4) -> Data Type Conversion19/1
  LegMedulla_A_L/20(Thermistor5) -> Data Type Conversion20/1
  LegMedulla_A_L/21(Amp1MeasuredCurrent) -> Data Type Conversion21/1
  LegMedulla_A_L/22(Amp2MeasuredCurrent) -> Data Type Conversion22/1
  LegMedulla_A_L/23(KneeForce1) -> Data Type Conversion23/1
  LegMedulla_A_L/24(KneeForce2) -> Data Type Conversion24/1
  [MedullaCmd3] -> LegMedulla_A_L/1(MedullaCmd)
  [Counter] -> LegMedulla_A_L/2(MedullaCounter)
  [MedullaCmd1] -> LegMedulla_A_R/1(MedullaCmd)
  [Counter] -> LegMedulla_A_R/2(MedullaCounter)
  LegMedulla_A_R/1(LegEncoder) -> Data Type Conversion49/1
  LegMedulla_A_R/2(MotorEncoder) -> Data Type Conversion50/1
  LegMedulla_A_R/3(ToeSensor) -> Data Type Conversion51/1
  LegMedulla_A_R/4(LimitSwitch) -> Data Type Conversion52/1
  LegMedulla_A_R/5(ID) -> Data Type Conversion53/1
  LegMedulla_A_R/6(State) -> Data Type Conversion54/1
  LegMedulla_A_R/7(Counter) -> Data Type Conversion55/1
  LegMedulla_A_R/8(ErrorFlags) -> Data Type Conversion56/1
  LegMedulla_A_R/9(IncEncoder) -> Data Type Conversion57/1
  LegMedulla_A_R/10(LegEncoderTimestamp) -> Data Type Conversion58/1
  LegMedulla_A_R/11(MotorEncoderTimestamp) -> Data Type Conversion59/1
  LegMedulla_A_R/12(IncEncoderTimestamp) -> Data Type Conversion60/1
  LegMedulla_A_R/13(MotorVoltage) -> Data Type Conversion61/1
  LegMedulla_A_R/14(LogicVoltage) -> Data Type Conversion62/1
  LegMedulla_A_R/15(Thermistor0) -> Data Type Conversion63/1
  LegMedulla_A_R/16(Thermistor1) -> Data Type Conversion64/1
  LegMedulla_A_R/17(Thermistor2) -> Data Type Conversion65/1
  LegMedulla_A_R/18(Thermistor3) -> Data Type Conversion66/1
  LegMedulla_A_R/19(Thermistor4) -> Data Type Conversion67/1
  LegMedulla_A_R/20(Thermistor5) -> Data Type Conversion68/1
  LegMedulla_A_R/21(Amp1MeasuredCurrent) -> Data Type Conversion69/1
  LegMedulla_A_R/22(Amp2MeasuredCurrent) -> Data Type Conversion70/1
  LegMedulla_A_R/23(KneeForce1) -> Data Type Conversion71/1
  LegMedulla_A_R/24(KneeForce2) -> Data Type Conversion72/1
  LegMedulla_B_L/1(LegEncoder) -> Data Type Conversion25/1
  LegMedulla_B_L/2(MotorEncoder) -> Data Type Conversion26/1
  LegMedulla_B_L/3(ToeSensor) -> Data Type Conversion27/1
  LegMedulla_B_L/4(LimitSwitch) -> Data Type Conversion28/1
  LegMedulla_B_L/5(ID) -> Data Type Conversion29/1
  LegMedulla_B_L/6(State) -> Data Type Conversion30/1
  LegMedulla_B_L/7(Counter) -> Data Type Conversion31/1
  LegMedulla_B_L/8(ErrorFlags) -> Data Type Conversion32/1
  LegMedulla_B_L/9(IncEncoder) -> Data Type Conversion33/1
  LegMedulla_B_L/10(LegEncoderTimestamp) -> Data Type Conversion34/1
  LegMedulla_B_L/11(MotorEncoderTimestamp) -> Data Type Conversion35/1
  LegMedulla_B_L/12(IncEncoderTimestamp) -> Data Type Conversion36/1
  LegMedulla_B_L/13(MotorVoltage) -> Data Type Conversion37/1
  LegMedulla_B_L/14(LogicVoltage) -> Data Type Conversion38/1
  LegMedulla_B_L/15(Thermistor0) -> Data Type Conversion39/1
  LegMedulla_B_L/16(Thermistor1) -> Data Type Conversion40/1
  LegMedulla_B_L/17(Thermistor2) -> Data Type Conversion41/1
  LegMedulla_B_L/18(Thermistor3) -> Data Type Conversion42/1
  LegMedulla_B_L/19(Thermistor4) -> Data Type Conversion43/1
  LegMedulla_B_L/20(Thermistor5) -> Data Type Conversion44/1
  LegMedulla_B_L/21(Amp1MeasuredCurrent) -> Data Type Conversion45/1
  LegMedulla_B_L/22(Amp2MeasuredCurrent) -> Data Type Conversion46/1
  LegMedulla_B_L/23(KneeForce1) -> Data Type Conversion47/1
  LegMedulla_B_L/24(KneeForce2) -> Data Type Conversion48/1
  [MedullaCmd4] -> LegMedulla_B_L/1(MedullaCmd)
  [Counter] -> LegMedulla_B_L/2(MedullaCounter)
  [MedullaCmd2] -> LegMedulla_B_R/1(MedullaCmd)
  [Counter] -> LegMedulla_B_R/2(MedullaCounter)
  LegMedulla_B_R/1(LegEncoder) -> Data Type Conversion73/1
  LegMedulla_B_R/2(MotorEncoder) -> Data Type Conversion74/1
  LegMedulla_B_R/3(ToeSensor) -> Data Type Conversion75/1
  LegMedulla_B_R/4(LimitSwitch) -> Data Type Conversion76/1
  LegMedulla_B_R/5(ID) -> Data Type Conversion77/1
  LegMedulla_B_R/6(State) -> Data Type Conversion78/1
  LegMedulla_B_R/7(Counter) -> Data Type Conversion79/1
  LegMedulla_B_R/8(ErrorFlags) -> Data Type Conversion80/1
  LegMedulla_B_R/9(IncEncoder) -> Data Type Conversion81/1
  LegMedulla_B_R/10(LegEncoderTimestamp) -> Data Type Conversion82/1
  LegMedulla_B_R/11(MotorEncoderTimestamp) -> Data Type Conversion83/1
  LegMedulla_B_R/12(IncEncoderTimestamp) -> Data Type Conversion84/1
  LegMedulla_B_R/13(MotorVoltage) -> Data Type Conversion85/1
  LegMedulla_B_R/14(LogicVoltage) -> Data Type Conversion86/1
  LegMedulla_B_R/15(Thermistor0) -> Data Type Conversion87/1
  LegMedulla_B_R/16(Thermistor1) -> Data Type Conversion88/1
  LegMedulla_B_R/17(Thermistor2) -> Data Type Conversion89/1
  LegMedulla_B_R/18(Thermistor3) -> Data Type Conversion90/1
  LegMedulla_B_R/19(Thermistor4) -> Data Type Conversion91/1
  LegMedulla_B_R/20(Thermistor5) -> Data Type Conversion92/1
  LegMedulla_B_R/21(Amp1MeasuredCurrent) -> Data Type Conversion93/1
  LegMedulla_B_R/22(Amp2MeasuredCurrent) -> Data Type Conversion94/1
  LegMedulla_B_R/23(KneeForce1) -> Data Type Conversion95/1
  LegMedulla_B_R/24(KneeForce2) -> Data Type Conversion96/1
  [MotorCmd3] -> Elmo Front Left/1(MotorCmd)
  Elmo Front Left/1(status) -> [Elmo_Front_Left]
  [MotorCmd1] -> Elmo Front Right/1(MotorCmd)
  Elmo Front Right/1(status) -> [Elmo_Front_Right]
  [MotorCmd4] -> Elmo Back Left/1(MotorCmd)
  Elmo Back Left/1(status) -> [Elmo_Back_Left]
  [MotorCmd2] -> Elmo Back Right/1(MotorCmd)
  Elmo Back Right/1(status) -> [Elmo_Back_Right]
  EtherCAT PDO Receive8/1 -> Data Type Conversion125/1
  [Counter] -> ?
  LegMedulla_B_R/25(counter send) -> Data Type Conversion124/1
  Data Type Conversion124/1 -> box 6 counter send/1
  LegMedulla_B_R/26(execution time) -> execution time/1
  Data Type Conversion125/1 -> box 6 counter receive/1

== system atrias_system_testing_delay/Ethercat Status Display ==
  Status : Inport
  Constant2 : Constant  Value=0  OutDataTypeStr=Inherit: Inherit via back propagation  SampleTime=-1
  Data Type Conversion{,1..6} (7 alike) : DataTypeConversion
  Demux : Demux  Outputs=6
  Discrete Filter2 : DiscreteFilter  Numerator="[0.001568334083281   0.001568334083281]"  Denominator="[1.000000000000000  -0.996863331833438]"  a0EqualsOne=on
  Mux2 : Mux  Inputs=3
  Mux3 : Mux  Inputs=6
  Scope 2 : slrtlib/Displays and Logging/Scope   scopeno=1  scopetype=Target  autostart=on  viewmode=Graphical rolling  formatstr='%f'  grid=on  ylimits=[0,0]  nosamples=10000  noprepostsamples=0  interleave=1  triggermode=FreeRun  triggersignal=1  trigsignalfromport=off  triggerlevel=0.0  triggerslope=Either  triggerscope=1  triggersample=0  filename=data.dat  mode=Lazy  writesize=512  autorestart=off  dynamicfilemode=off  maxwritefilesize=512*1024^2
  Scope 3 : slrtlib/Displays and Logging/Scope   scopeno=3  scopetype=Target  autostart=on  viewmode=Numerical  formatstr='%15.6f'  grid=on  ylimits=[0,0]  nosamples=100  noprepostsamples=0  interleave=1  triggermode=FreeRun  triggersignal=1  trigsignalfromport=off  triggerlevel=0.0  triggerslope=Either  triggerscope=1  triggersample=0  filename=data.dat  mode=Lazy  writesize=512  autorestart=off  dynamicfilemode=off  maxwritefilesize=512*1024^2
  wires:
  Status/1 -> Demux/1
  Demux/4 -> Discrete Filter2/1, Mux2/1
  Discrete Filter2/1 -> Data Type Conversion/1
  Mux2/1 -> Scope 2/1
  Constant2/1 -> Data Type Conversion4/1
  Data Type Conversion4/1 -> Mux2/3
  Mux3/1 -> Scope 3/1
  Data Type Conversion/1 -> Mux3/4, Mux2/2  "MasterRefToClockDiff"
  Data Type Conversion1/1 -> Mux3/1  "ErrVal"
  Data Type Conversion2/1 -> Mux3/2  "MasterState"
  Data Type Conversion3/1 -> Mux3/3  "DCErrVal"
  Data Type Conversion5/1 -> Mux3/5  "DCInitState"
  Data Type Conversion6/1 -> Mux3/6  "RefClockToSlaveDiff"
  Demux/1 -> Data Type Conversion1/1  "ErrVal"
  Demux/2 -> Data Type Conversion2/1  "MasterState"
  Demux/3 -> Data Type Conversion3/1  "DCErrVal"
  Demux/5 -> Data Type Conversion5/1  "DCInitState"
  Demux/6 -> Data Type Conversion6/1  "RefClockToSlaveDiff"

== system atrias_system_testing_delay/Start Controller ==
  note: Input Order:
      |
      | backR
      | frontR
      | latR
      | backL
      | frontL
      | latL
  is_run_cmd : Inport  OutDataTypeStr=boolean  PortDimensions=1
  tau_cmd_in [Nm] x6 : Inport  Port=2
  Current Time : Clock
  Enabled time : Sum  Inputs=-+
  Hold Start Time : Subsystem  TreatAsAtomicUnit=on
  Lateral Motor Saturation : Saturate  UpperLimit=HIP_MTR_MAX_TORQUE  LowerLimit=-HIP_MTR_MAX_TORQUE
      settings: AttributesFormatString=Top: %<UpperLimit>\nBottom: %<LowerLimit>
  NOT : Logic  Operator=NOT  IconShape=distinctive  AllPortsSameDT=off  OutDataTypeStr=boolean
  Ramp Rate (Units/sec) : Gain  Gain=.25
  Sagittal Motor Saturation : Saturate  UpperLimit=LEG_MTR_MAX_TORQUE  LowerLimit=-LEG_MTR_MAX_TORQUE
      settings: AttributesFormatString=Top: %<UpperLimit>\nBottom: %<LowerLimit>
  Scaling Factor : Saturate  UpperLimit=1  LowerLimit=0
  Selector : Selector  InputPortWidth=6  Indices=[1 2 4 5 6 3]
  Selector1 : Selector  InputPortWidth=6  Indices=[1 2 3 4]
  Selector2 : Selector  InputPortWidth=6  Indices=[5 6]
  Separated to Tau : Selector  InputPortWidth=6  Indices=[1 2 6 3 4 5]
  Startup Tau Ramp : Product
  Sum : Sum  Inputs=|-+
  Vector Concatenate : Concatenate
  is_start_done_cmp : RelationalOperator  Operator=>  OutDataTypeStr=boolean
  tau_cmd_out [Nm] x6 : Outport  OutDataTypeStr=double  PortDimensions=6
  is_start_done : Outport  Port=2
  wires:
  NOT/1 -> Hold Start Time/Enable
  is_run_cmd/1 -> NOT/1
  Current Time/1 -> Enabled time/2, Hold Start Time/1(Time In)
  Hold Start Time/1(Time Out) -> Enabled time/1
  Enabled time/1 -> Ramp Rate (Units/sec)/1
  Ramp Rate (Units/sec)/1 -> Scaling Factor/1, Sum/2
  Scaling Factor/1 -> is_start_done_cmp/2, Startup Tau Ramp/1
  Startup Tau Ramp/1 -> tau_cmd_out [Nm] x6/1
  Selector2/1 -> Lateral Motor Saturation/1  "lateral"
  Selector1/1 -> Sagittal Motor Saturation/1  "sagittal"
  tau_cmd_in [Nm] x6/1 -> Selector/1
  Selector/1 -> Selector1/1, Selector2/1
  Sagittal Motor Saturation/1 -> Vector Concatenate/1
  Lateral Motor Saturation/1 -> Vector Concatenate/2
  Vector Concatenate/1 -> Separated to Tau/1
  Separated to Tau/1 -> Startup Tau Ramp/2
  Sum/1 -> is_start_done_cmp/1
  is_start_done_cmp/1 -> is_start_done/1
